simulink model "QPSK"  (R2021a)
settings: Solver=VariableStepAuto  StartTime=0.0  StopTime=0.002  RelTol=1e-3
libraries: dsparch4 x3, dspsigops x2, commchan3 x1, commrandsrc3 x1, commutil2 x1, commsink2 x1, dspindex x1
settings Model: Creator=MrCai  LastModifiedBy=MrCai

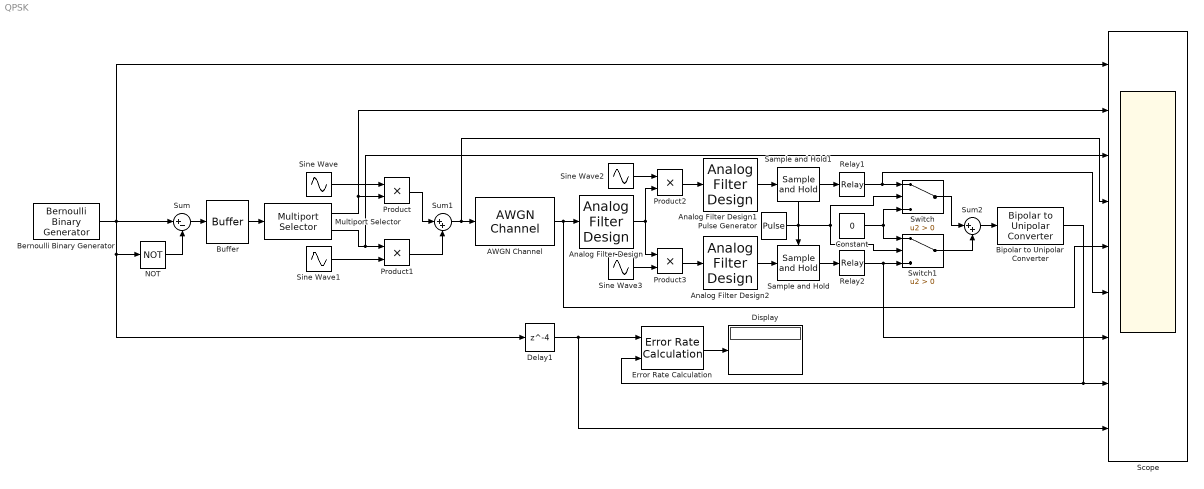
== system QPSK ==
  AWGN Channel : commchan3/AWGN Channel  InputProcessing=Columns as channels (frame based)  seed=67  noiseMode="Signal to noise ratio  (SNR)"  EbNodB=10  EsNodB=10  SNRdB=10  bitsPerSym=1  Ps=1  Tsym=1  variance=1
  Analog Filter Design : dsparch4/Analog Filter Design  method=Butterworth  filttype=Bandpass  N=8  Wlo=2*pi*90*1000  Whi=2*pi*110*1000  Rp=2  Rs=40
  Analog Filter Design1 : dsparch4/Analog Filter Design  method=Butterworth  filttype=Lowpass  N=8  Wlo=2*pi*10*1000  Whi=80  Rp=2  Rs=40
  Analog Filter Design2 : dsparch4/Analog Filter Design  method=Butterworth  filttype=Lowpass  N=8  Wlo=2*pi*10*1000  Whi=80  Rp=2  Rs=40
  Bernoulli Binary Generator : commrandsrc3/Bernoulli Binary Generator  ProbabilityOfZero=0.5  SeedSource=Auto  Seed=0  SampleTime=1/10000  SamplesPerFrame=1  OutputDataType=double  SimulateUsing=Interpreted execution
  Bipolar to Unipolar Converter : commutil2/Bipolar to Unipolar Converter  M=2  polarity=Positive  dataType=Inherit via internal rule
      settings: SourceProductBaseCode=CM
  Buffer : Buffer  N=2  OutputFrames=off
  Constant : Constant  Value=0
  Delay1 : Delay  DelayLength=4
  Display : Display
  Error Rate Calculation : commsink2/Error Rate Calculation  N=0  st_delay=0  cp_mode=Entire frame  subframe=[]  PMode=Port  WsName=ErrorVec  RsMode2=off  stop=off  numErr=100  maxBits=1e6
  Multiport Selector : dspindex/Multiport Selector  rowsOrCols=Rows  idxCellArray={1,2}  idxErrMode=Clip Index
  NOT : Logic  Operator=NOT  IconShape=distinctive  AllPortsSameDT=off  OutDataTypeStr=boolean
  Product{,1..3} (4 alike) : Product
  Pulse Generator : DiscretePulseGenerator  SampleTime=1/10000
  Relay1 : Relay  OnSwitchValue=0.2  OffSwitchValue=0.2  OffOutputValue=-1
  Relay2 : Relay  OnSwitchValue=0.2  OffSwitchValue=0.2  OffOutputValue=-1
  Sample and Hold : dspsigops/Sample and Hold  trig=Rising edge  initCond=0  latchinput=off
  Sample and Hold1 : dspsigops/Sample and Hold  trig=Rising edge  initCond=0  latchinput=off
  Scope : Scope  NumInputPorts=9
  Sine Wave : Sin  Frequency=2*pi*100*1000  Phase=pi/2  SampleTime=1/1000000
  Sine Wave1 : Sin  Frequency=2*pi*100*1000  Phase=pi  SampleTime=1/1000000
  Sine Wave2 : Sin  Frequency=2*pi*100*1000  Phase=pi/2  SampleTime=1/1000000
  Sine Wave3 : Sin  Frequency=2*pi*100*1000  Phase=pi  SampleTime=1/1000000
  Sum : Sum  Inputs=|+-
  Sum1 : Sum  Inputs=|++
  Sum2 : Sum  Inputs=|++
  Switch : Switch  Criteria=u2 > Threshold
  Switch1 : Switch  Criteria=u2 > Threshold
  wires:
  Buffer/1 -> Multiport Selector/1
  Multiport Selector/1 -> Product/2, Scope/2
  Sine Wave/1 -> Product/1
  Sine Wave1/1 -> Product1/2
  Product/1 -> Sum1/1
  Product1/1 -> Sum1/2
  Sum1/1 -> Scope/4, AWGN Channel/1
  AWGN Channel/1 -> Scope/5, Analog Filter Design/1
  Sine Wave3/1 -> Product3/2
  Sine Wave2/1 -> Product2/1
  Analog Filter Design/1 -> Product2/2, Product3/1
  Bernoulli Binary Generator/1 -> Delay1/1, NOT/1, Scope/1, Sum/1
  Sum/1 -> Buffer/1
  NOT/1 -> Sum/2
  Product2/1 -> Analog Filter Design1/1
  Product3/1 -> Analog Filter Design2/1
  Multiport Selector/2 -> Scope/3, Product1/1
  Error Rate Calculation/1 -> Display/1
  Delay1/1 -> Scope/9, Error Rate Calculation/1
  Analog Filter Design1/1 -> Sample and Hold1/1
  Analog Filter Design2/1 -> Sample and Hold/1
  Sample and Hold/1 -> Relay2/1
  Sample and Hold1/1 -> Relay1/1
  Pulse Generator/1 -> Switch1/2, Switch/2, Sample and Hold/Trigger, Sample and Hold1/Trigger
  Constant/1 -> Switch1/1, Switch/3
  Relay2/1 -> Scope/7, Switch1/3
  Relay1/1 -> Scope/6, Switch/1
  Switch/1 -> Sum2/1
  Switch1/1 -> Sum2/2
  Sum2/1 -> Bipolar to Unipolar Converter/1
  Bipolar to Unipolar Converter/1 -> Error Rate Calculation/2, Scope/8
